simulink model "Pokus08_Display_16x1"  (Simulink 8.1)
settings: Solver=FixedStepDiscrete  StartTime=0.0  StopTime=10.0  RelTol=1e-3
libraries: simulink_extras x1, Displays_Lib x1, Computer_Library x1
settings Model: Creator=uzivatel  LastModifiedBy=uzivatel
settings DataIOCC: SignalLoggingSaveFormat=Dataset
settings OptimizationCC: ExpressionDepthLimit=128
settings DebuggingCC: FcnCallInpInsideContextMsg=EnableAllAsError
settings GRTTargetCC: CombineOutputUpdateFcns=on  GRTInterface=off

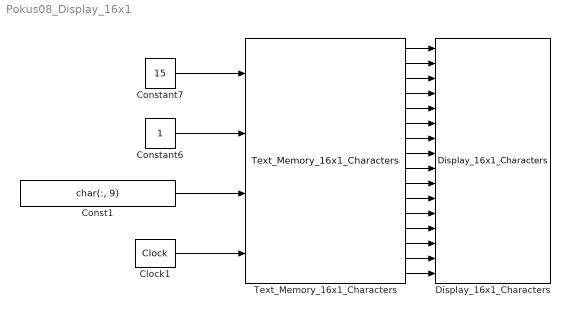
== system Pokus08_Display_16x1 ==
  Clock1 : simulink_extras/Flip Flops/Clock  period=1
  Const1 : Constant  Value=char(:, 9)  OutDataTypeStr=uint8
  Constant6 : Constant  OutDataTypeStr=uint8
  Constant7 : Constant  Value=15  OutDataTypeStr=uint8
  Display_16x1_Characters : Displays_Lib/Displays_Lib/Display_16x1_Characters
  Text_Memory_16x1_Characters : Computer_Library/Text_Memory_16x1_Characters
  wires:
  Constant7/1 -> Text_Memory_16x1_Characters/1
  Constant6/1 -> Text_Memory_16x1_Characters/2
  Const1/1 -> Text_Memory_16x1_Characters/3
  Clock1/1 -> Text_Memory_16x1_Characters/4
  Text_Memory_16x1_Characters/1 -> Display_16x1_Characters/1
  Text_Memory_16x1_Characters/2 -> Display_16x1_Characters/2
  Text_Memory_16x1_Characters/3 -> Display_16x1_Characters/3
  Text_Memory_16x1_Characters/4 -> Display_16x1_Characters/4
  Text_Memory_16x1_Characters/5 -> Display_16x1_Characters/5
  Text_Memory_16x1_Characters/6 -> Display_16x1_Characters/6
  Text_Memory_16x1_Characters/7 -> Display_16x1_Characters/7
  Text_Memory_16x1_Characters/8 -> Display_16x1_Characters/8
  Text_Memory_16x1_Characters/9 -> Display_16x1_Characters/9
  Text_Memory_16x1_Characters/10 -> Display_16x1_Characters/10
  Text_Memory_16x1_Characters/11 -> Display_16x1_Characters/11
  Text_Memory_16x1_Characters/12 -> Display_16x1_Characters/12
  Text_Memory_16x1_Characters/13 -> Display_16x1_Characters/13
  Text_Memory_16x1_Characters/14 -> Display_16x1_Characters/14
  Text_Memory_16x1_Characters/15 -> Display_16x1_Characters/15
  Text_Memory_16x1_Characters/16 -> Display_16x1_Characters/16
